simulink model "Simulink"  (R2020b)
settings: Solver=VariableStepAuto  StartTime=0.0  StopTime=11.2395  RelTol=1e-3
values from neighbouring files (symbols this model uses):
  alpha_0 = 1    [Main.m]
  b = 10    [Main.m]
  beta = 3    [Main.m]
  beta_0 = 1    [Main.m]
  c1 = rand(8,8)-0.5    [Main.m]
  c2 = rand(8,8)-0.5    [Main.m]
  c3 = rand(8,8)-0.5    [Main.m]
  c4 = rand(8,8)-0.5    [Main.m]
  delta_0 = 1    [Main.m]
  Gamma = 3    [Main.m]
  gamma = 0.1    [Main.m]
  h1_x = 5    [Main.m]
  h1_y = 5    [Main.m]
  h2_x = -5    [Main.m]
  h2_y = 5    [Main.m]
  h3_x = -5    [Main.m]
  h3_y = -5    [Main.m]
  h4_x = 5    [Main.m]
  h4_y = -5    [Main.m]
  kapa = 3    [Main.m]
  ki = diag([150,150])    [Main.m]
  kp = 20    [Main.m]
  L = full(laplacian(G))    [Main.m]
  m = 3    [Main.m]
  obs_x = 40    [Main.m]
  obs_y = 0    [Main.m]
  R = 5    [Main.m]
  r = 2    [Main.m]
  R_reg = 15    [Main.m]
  region_x = 80    [Main.m]
  region_y = 0    [Main.m]
  row_0 = 0    [Main.m]
  WL_0 = rand(number_of_neurons,1)*2    [Main.m]
  WR_0 = rand(number_of_neurons,1)*2    [Main.m]
  x1_0 = 1    [Main.m]
  x1_dot_0 = 0    [Main.m]
  x2_0 = 1    [Main.m]
  x2_dot_0 = 0    [Main.m]
  x3_0 = 1    [Main.m]
  x3_dot_0 = 0    [Main.m]
  x4_0 = 1    [Main.m]
  x4_dot_0 = 0    [Main.m]
  y1_0 = 9    [Main.m]
  y1_dot_0 = 0    [Main.m]
  y2_0 = 3    [Main.m]
  y2_dot_0 = 0    [Main.m]
  y3_0 = -3    [Main.m]
  y3_dot_0 = 0    [Main.m]
  y4_0 = -9    [Main.m]
  y4_dot_0 = 0    [Main.m]
(part 2 of 2)

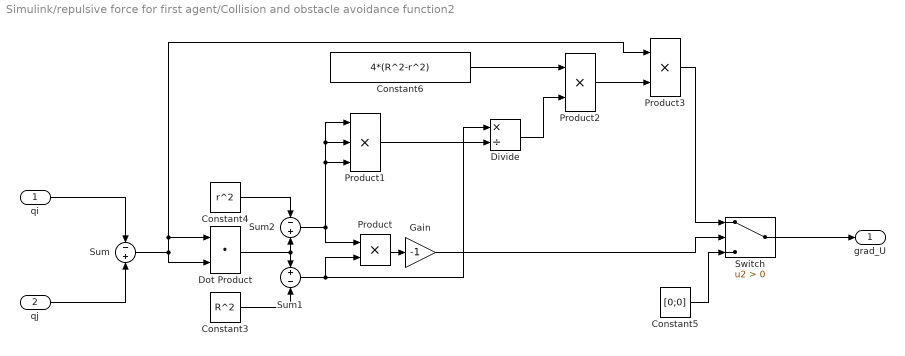
== system Simulink/repulsive force for first agent/Collision and obstacle avoidance function2 ==
  qi : Inport
  qj : Inport  Port=2
  Constant3 : Constant  Value=R^2
  Constant4 : Constant  Value=r^2
  Constant5 : Constant  Value=[0;0]
  Constant6 : Constant  Value=4*(R^2-r^2)
  Divide : Product  Inputs=*/
  Dot Product : DotProduct  InputSameDT=on  OutDataTypeStr=Inherit: Inherit via internal rule
  Gain : Gain  Gain=-1
  Product : Product
  Product1 : Product  Inputs=3
  Product2 : Product
  Product3 : Product
  Sum : Sum  Inputs=-+
  Sum1 : Sum  Inputs=+-
  Sum2 : Sum  Inputs=-+
  Switch : Switch  Criteria=u2 > Threshold
  grad_U : Outport
  wires:
  Sum1/1 -> Divide/1, Product/2
  Sum2/1 -> Product1/1, Product1/2, Product1/3, Product/1
  qi/1 -> Sum/1
  Dot Product/1 -> Sum2/2, Sum1/1
  Product1/1 -> Divide/2
  Constant5/1 -> Switch/3
  Constant4/1 -> Sum2/1
  Divide/1 -> Product2/2
  Constant3/1 -> Sum1/2
  Sum/1 -> Product3/1, Dot Product/1, Dot Product/2
  Product/1 -> Gain/1
  Gain/1 -> Switch/2
  Constant6/1 -> Product2/1
  Product3/1 -> Switch/1
  Product2/1 -> Product3/2
  Switch/1 -> grad_U/1
  qj/1 -> Sum/2

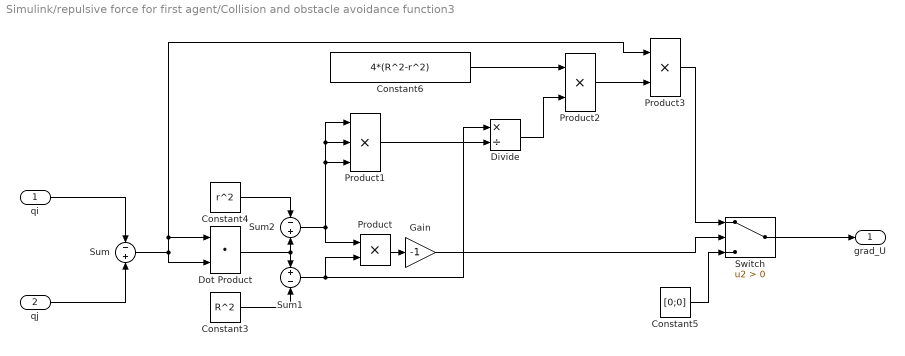
== system Simulink/repulsive force for first agent/Collision and obstacle avoidance function3 ==
  qi : Inport
  qj : Inport  Port=2
  Constant3 : Constant  Value=R^2
  Constant4 : Constant  Value=r^2
  Constant5 : Constant  Value=[0;0]
  Constant6 : Constant  Value=4*(R^2-r^2)
  Divide : Product  Inputs=*/
  Dot Product : DotProduct  InputSameDT=on  OutDataTypeStr=Inherit: Inherit via internal rule
  Gain : Gain  Gain=-1
  Product : Product
  Product1 : Product  Inputs=3
  Product2 : Product
  Product3 : Product
  Sum : Sum  Inputs=-+
  Sum1 : Sum  Inputs=+-
  Sum2 : Sum  Inputs=-+
  Switch : Switch  Criteria=u2 > Threshold
  grad_U : Outport
  wires:
  qj/1 -> Sum/2
  Switch/1 -> grad_U/1
  Product2/1 -> Product3/2
  Product3/1 -> Switch/1
  Constant6/1 -> Product2/1
  Gain/1 -> Switch/2
  Product/1 -> Gain/1
  Sum/1 -> Dot Product/2, Dot Product/1, Product3/1
  Constant3/1 -> Sum1/2
  Divide/1 -> Product2/2
  Constant4/1 -> Sum2/1
  Constant5/1 -> Switch/3
  Product1/1 -> Divide/2
  Dot Product/1 -> Sum1/1, Sum2/2
  qi/1 -> Sum/1
  Sum2/1 -> Product/1, Product1/3, Product1/2, Product1/1
  Sum1/1 -> Product/2, Divide/1

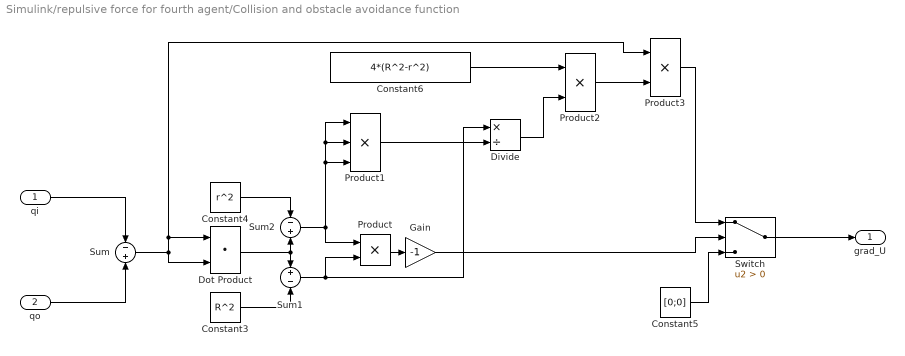
== system Simulink/repulsive force for fourth agent/Collision and obstacle avoidance function ==
  qi : Inport
  qo : Inport  Port=2
  Constant3 : Constant  Value=R^2
  Constant4 : Constant  Value=r^2
  Constant5 : Constant  Value=[0;0]
  Constant6 : Constant  Value=4*(R^2-r^2)
  Divide : Product  Inputs=*/
  Dot Product : DotProduct  InputSameDT=on  OutDataTypeStr=Inherit: Inherit via internal rule
  Gain : Gain  Gain=-1
  Product : Product
  Product1 : Product  Inputs=3
  Product2 : Product
  Product3 : Product
  Sum : Sum  Inputs=-+
  Sum1 : Sum  Inputs=+-
  Sum2 : Sum  Inputs=-+
  Switch : Switch  Criteria=u2 > Threshold
  grad_U : Outport
  wires:
  Sum1/1 -> Divide/1, Product/2
  Sum2/1 -> Product1/1, Product1/2, Product1/3, Product/1
  qi/1 -> Sum/1
  Dot Product/1 -> Sum2/2, Sum1/1
  Product1/1 -> Divide/2
  Constant5/1 -> Switch/3
  Constant4/1 -> Sum2/1
  Divide/1 -> Product2/2
  Constant3/1 -> Sum1/2
  Sum/1 -> Product3/1, Dot Product/1, Dot Product/2
  Product/1 -> Gain/1
  Gain/1 -> Switch/2
  Constant6/1 -> Product2/1
  Product3/1 -> Switch/1
  Product2/1 -> Product3/2
  Switch/1 -> grad_U/1
  qo/1 -> Sum/2

== system Simulink/repulsive force for fourth agent/Collision and obstacle avoidance function1 ==
  qi : Inport
  qj : Inport  Port=2
  Constant3 : Constant  Value=R^2
  Constant4 : Constant  Value=r^2
  Constant5 : Constant  Value=[0;0]
  Constant6 : Constant  Value=4*(R^2-r^2)
  Divide : Product  Inputs=*/
  Dot Product : DotProduct  InputSameDT=on  OutDataTypeStr=Inherit: Inherit via internal rule
  Gain : Gain  Gain=-1
  Product : Product
  Product1 : Product  Inputs=3
  Product2 : Product
  Product3 : Product
  Sum : Sum  Inputs=-+
  Sum1 : Sum  Inputs=+-
  Sum2 : Sum  Inputs=-+
  Switch : Switch  Criteria=u2 > Threshold
  grad_U : Outport
  wires:
  qj/1 -> Sum/2
  Switch/1 -> grad_U/1
  Product2/1 -> Product3/2
  Product3/1 -> Switch/1
  Constant6/1 -> Product2/1
  Gain/1 -> Switch/2
  Product/1 -> Gain/1
  Sum/1 -> Dot Product/2, Dot Product/1, Product3/1
  Constant3/1 -> Sum1/2
  Divide/1 -> Product2/2
  Constant4/1 -> Sum2/1
  Constant5/1 -> Switch/3
  Product1/1 -> Divide/2
  Dot Product/1 -> Sum1/1, Sum2/2
  qi/1 -> Sum/1
  Sum2/1 -> Product/1, Product1/3, Product1/2, Product1/1
  Sum1/1 -> Product/2, Divide/1

== system Simulink/repulsive force for fourth agent/Collision and obstacle avoidance function2 ==
  qi : Inport
  qj : Inport  Port=2
  Constant3 : Constant  Value=R^2
  Constant4 : Constant  Value=r^2
  Constant5 : Constant  Value=[0;0]
  Constant6 : Constant  Value=4*(R^2-r^2)
  Divide : Product  Inputs=*/
  Dot Product : DotProduct  InputSameDT=on  OutDataTypeStr=Inherit: Inherit via internal rule
  Gain : Gain  Gain=-1
  Product : Product
  Product1 : Product  Inputs=3
  Product2 : Product
  Product3 : Product
  Sum : Sum  Inputs=-+
  Sum1 : Sum  Inputs=+-
  Sum2 : Sum  Inputs=-+
  Switch : Switch  Criteria=u2 > Threshold
  grad_U : Outport
  wires:
  Sum1/1 -> Divide/1, Product/2
  Sum2/1 -> Product1/1, Product1/2, Product1/3, Product/1
  qi/1 -> Sum/1
  Dot Product/1 -> Sum2/2, Sum1/1
  Product1/1 -> Divide/2
  Constant5/1 -> Switch/3
  Constant4/1 -> Sum2/1
  Divide/1 -> Product2/2
  Constant3/1 -> Sum1/2
  Sum/1 -> Product3/1, Dot Product/1, Dot Product/2
  Product/1 -> Gain/1
  Gain/1 -> Switch/2
  Constant6/1 -> Product2/1
  Product3/1 -> Switch/1
  Product2/1 -> Product3/2
  Switch/1 -> grad_U/1
  qj/1 -> Sum/2

== system Simulink/repulsive force for fourth agent/Collision and obstacle avoidance function3 ==
  qi : Inport
  qj : Inport  Port=2
  Constant3 : Constant  Value=R^2
  Constant4 : Constant  Value=r^2
  Constant5 : Constant  Value=[0;0]
  Constant6 : Constant  Value=4*(R^2-r^2)
  Divide : Product  Inputs=*/
  Dot Product : DotProduct  InputSameDT=on  OutDataTypeStr=Inherit: Inherit via internal rule
  Gain : Gain  Gain=-1
  Product : Product
  Product1 : Product  Inputs=3
  Product2 : Product
  Product3 : Product
  Sum : Sum  Inputs=-+
  Sum1 : Sum  Inputs=+-
  Sum2 : Sum  Inputs=-+
  Switch : Switch  Criteria=u2 > Threshold
  grad_U : Outport
  wires:
  qj/1 -> Sum/2
  Switch/1 -> grad_U/1
  Product2/1 -> Product3/2
  Product3/1 -> Switch/1
  Constant6/1 -> Product2/1
  Gain/1 -> Switch/2
  Product/1 -> Gain/1
  Sum/1 -> Dot Product/2, Dot Product/1, Product3/1
  Constant3/1 -> Sum1/2
  Divide/1 -> Product2/2
  Constant4/1 -> Sum2/1
  Constant5/1 -> Switch/3
  Product1/1 -> Divide/2
  Dot Product/1 -> Sum1/1, Sum2/2
  qi/1 -> Sum/1
  Sum2/1 -> Product/1, Product1/3, Product1/2, Product1/1
  Sum1/1 -> Product/2, Divide/1

== system Simulink/repulsive force for second agent/Collision and obstacle avoidance function ==
  qi : Inport
  qo : Inport  Port=2
  Constant3 : Constant  Value=R^2
  Constant4 : Constant  Value=r^2
  Constant5 : Constant  Value=[0;0]
  Constant6 : Constant  Value=4*(R^2-r^2)
  Divide : Product  Inputs=*/
  Dot Product : DotProduct  InputSameDT=on  OutDataTypeStr=Inherit: Inherit via internal rule
  Gain : Gain  Gain=-1
  Product : Product
  Product1 : Product  Inputs=3
  Product2 : Product
  Product3 : Product
  Sum : Sum  Inputs=-+
  Sum1 : Sum  Inputs=+-
  Sum2 : Sum  Inputs=-+
  Switch : Switch  Criteria=u2 > Threshold
  grad_U : Outport
  wires:
  qo/1 -> Sum/2
  Switch/1 -> grad_U/1
  Product2/1 -> Product3/2
  Product3/1 -> Switch/1
  Constant6/1 -> Product2/1
  Gain/1 -> Switch/2
  Product/1 -> Gain/1
  Sum/1 -> Dot Product/2, Dot Product/1, Product3/1
  Constant3/1 -> Sum1/2
  Divide/1 -> Product2/2
  Constant4/1 -> Sum2/1
  Constant5/1 -> Switch/3
  Product1/1 -> Divide/2
  Dot Product/1 -> Sum1/1, Sum2/2
  qi/1 -> Sum/1
  Sum2/1 -> Product/1, Product1/3, Product1/2, Product1/1
  Sum1/1 -> Product/2, Divide/1

== system Simulink/repulsive force for second agent/Collision and obstacle avoidance function1 ==
  qi : Inport
  qj : Inport  Port=2
  Constant3 : Constant  Value=R^2
  Constant4 : Constant  Value=r^2
  Constant5 : Constant  Value=[0;0]
  Constant6 : Constant  Value=4*(R^2-r^2)
  Divide : Product  Inputs=*/
  Dot Product : DotProduct  InputSameDT=on  OutDataTypeStr=Inherit: Inherit via internal rule
  Gain : Gain  Gain=-1
  Product : Product
  Product1 : Product  Inputs=3
  Product2 : Product
  Product3 : Product
  Sum : Sum  Inputs=-+
  Sum1 : Sum  Inputs=+-
  Sum2 : Sum  Inputs=-+
  Switch : Switch  Criteria=u2 > Threshold
  grad_U : Outport
  wires:
  Sum1/1 -> Divide/1, Product/2
  Sum2/1 -> Product1/1, Product1/2, Product1/3, Product/1
  qi/1 -> Sum/1
  Dot Product/1 -> Sum2/2, Sum1/1
  Product1/1 -> Divide/2
  Constant5/1 -> Switch/3
  Constant4/1 -> Sum2/1
  Divide/1 -> Product2/2
  Constant3/1 -> Sum1/2
  Sum/1 -> Product3/1, Dot Product/1, Dot Product/2
  Product/1 -> Gain/1
  Gain/1 -> Switch/2
  Constant6/1 -> Product2/1
  Product3/1 -> Switch/1
  Product2/1 -> Product3/2
  Switch/1 -> grad_U/1
  qj/1 -> Sum/2

== system Simulink/repulsive force for second agent/Collision and obstacle avoidance function2 ==
  qi : Inport
  qj : Inport  Port=2
  Constant3 : Constant  Value=R^2
  Constant4 : Constant  Value=r^2
  Constant5 : Constant  Value=[0;0]
  Constant6 : Constant  Value=4*(R^2-r^2)
  Divide : Product  Inputs=*/
  Dot Product : DotProduct  InputSameDT=on  OutDataTypeStr=Inherit: Inherit via internal rule
  Gain : Gain  Gain=-1
  Product : Product
  Product1 : Product  Inputs=3
  Product2 : Product
  Product3 : Product
  Sum : Sum  Inputs=-+
  Sum1 : Sum  Inputs=+-
  Sum2 : Sum  Inputs=-+
  Switch : Switch  Criteria=u2 > Threshold
  grad_U : Outport
  wires:
  qj/1 -> Sum/2
  Switch/1 -> grad_U/1
  Product2/1 -> Product3/2
  Product3/1 -> Switch/1
  Constant6/1 -> Product2/1
  Gain/1 -> Switch/2
  Product/1 -> Gain/1
  Sum/1 -> Dot Product/2, Dot Product/1, Product3/1
  Constant3/1 -> Sum1/2
  Divide/1 -> Product2/2
  Constant4/1 -> Sum2/1
  Constant5/1 -> Switch/3
  Product1/1 -> Divide/2
  Dot Product/1 -> Sum1/1, Sum2/2
  qi/1 -> Sum/1
  Sum2/1 -> Product/1, Product1/3, Product1/2, Product1/1
  Sum1/1 -> Product/2, Divide/1

== system Simulink/repulsive force for second agent/Collision and obstacle avoidance function3 ==
  qi : Inport
  qj : Inport  Port=2
  Constant3 : Constant  Value=R^2
  Constant4 : Constant  Value=r^2
  Constant5 : Constant  Value=[0;0]
  Constant6 : Constant  Value=4*(R^2-r^2)
  Divide : Product  Inputs=*/
  Dot Product : DotProduct  InputSameDT=on  OutDataTypeStr=Inherit: Inherit via internal rule
  Gain : Gain  Gain=-1
  Product : Product
  Product1 : Product  Inputs=3
  Product2 : Product
  Product3 : Product
  Sum : Sum  Inputs=-+
  Sum1 : Sum  Inputs=+-
  Sum2 : Sum  Inputs=-+
  Switch : Switch  Criteria=u2 > Threshold
  grad_U : Outport
  wires:
  Sum1/1 -> Divide/1, Product/2
  Sum2/1 -> Product1/1, Product1/2, Product1/3, Product/1
  qi/1 -> Sum/1
  Dot Product/1 -> Sum2/2, Sum1/1
  Product1/1 -> Divide/2
  Constant5/1 -> Switch/3
  Constant4/1 -> Sum2/1
  Divide/1 -> Product2/2
  Constant3/1 -> Sum1/2
  Sum/1 -> Product3/1, Dot Product/1, Dot Product/2
  Product/1 -> Gain/1
  Gain/1 -> Switch/2
  Constant6/1 -> Product2/1
  Product3/1 -> Switch/1
  Product2/1 -> Product3/2
  Switch/1 -> grad_U/1
  qj/1 -> Sum/2

== system Simulink/repulsive force for third agent/Collision and obstacle avoidance function ==
  qi : Inport
  qo : Inport  Port=2
  Constant3 : Constant  Value=R^2
  Constant4 : Constant  Value=r^2
  Constant5 : Constant  Value=[0;0]
  Constant6 : Constant  Value=4*(R^2-r^2)
  Divide : Product  Inputs=*/
  Dot Product : DotProduct  InputSameDT=on  OutDataTypeStr=Inherit: Inherit via internal rule
  Gain : Gain  Gain=-1
  Product : Product
  Product1 : Product  Inputs=3
  Product2 : Product
  Product3 : Product
  Sum : Sum  Inputs=-+
  Sum1 : Sum  Inputs=+-
  Sum2 : Sum  Inputs=-+
  Switch : Switch  Criteria=u2 > Threshold
  grad_U : Outport
  wires:
  qo/1 -> Sum/2
  Switch/1 -> grad_U/1
  Product2/1 -> Product3/2
  Product3/1 -> Switch/1
  Constant6/1 -> Product2/1
  Gain/1 -> Switch/2
  Product/1 -> Gain/1
  Sum/1 -> Dot Product/2, Dot Product/1, Product3/1
  Constant3/1 -> Sum1/2
  Divide/1 -> Product2/2
  Constant4/1 -> Sum2/1
  Constant5/1 -> Switch/3
  Product1/1 -> Divide/2
  Dot Product/1 -> Sum1/1, Sum2/2
  qi/1 -> Sum/1
  Sum2/1 -> Product/1, Product1/3, Product1/2, Product1/1
  Sum1/1 -> Product/2, Divide/1

== system Simulink/repulsive force for third agent/Collision and obstacle avoidance function1 ==
  qi : Inport
  qj : Inport  Port=2
  Constant3 : Constant  Value=R^2
  Constant4 : Constant  Value=r^2
  Constant5 : Constant  Value=[0;0]
  Constant6 : Constant  Value=4*(R^2-r^2)
  Divide : Product  Inputs=*/
  Dot Product : DotProduct  InputSameDT=on  OutDataTypeStr=Inherit: Inherit via internal rule
  Gain : Gain  Gain=-1
  Product : Product
  Product1 : Product  Inputs=3
  Product2 : Product
  Product3 : Product
  Sum : Sum  Inputs=-+
  Sum1 : Sum  Inputs=+-
  Sum2 : Sum  Inputs=-+
  Switch : Switch  Criteria=u2 > Threshold
  grad_U : Outport
  wires:
  Sum1/1 -> Divide/1, Product/2
  Sum2/1 -> Product1/1, Product1/2, Product1/3, Product/1
  qi/1 -> Sum/1
  Dot Product/1 -> Sum2/2, Sum1/1
  Product1/1 -> Divide/2
  Constant5/1 -> Switch/3
  Constant4/1 -> Sum2/1
  Divide/1 -> Product2/2
  Constant3/1 -> Sum1/2
  Sum/1 -> Product3/1, Dot Product/1, Dot Product/2
  Product/1 -> Gain/1
  Gain/1 -> Switch/2
  Constant6/1 -> Product2/1
  Product3/1 -> Switch/1
  Product2/1 -> Product3/2
  Switch/1 -> grad_U/1
  qj/1 -> Sum/2

== system Simulink/repulsive force for third agent/Collision and obstacle avoidance function2 ==
  qi : Inport
  qj : Inport  Port=2
  Constant3 : Constant  Value=R^2
  Constant4 : Constant  Value=r^2
  Constant5 : Constant  Value=[0;0]
  Constant6 : Constant  Value=4*(R^2-r^2)
  Divide : Product  Inputs=*/
  Dot Product : DotProduct  InputSameDT=on  OutDataTypeStr=Inherit: Inherit via internal rule
  Gain : Gain  Gain=-1
  Product : Product
  Product1 : Product  Inputs=3
  Product2 : Product
  Product3 : Product
  Sum : Sum  Inputs=-+
  Sum1 : Sum  Inputs=+-
  Sum2 : Sum  Inputs=-+
  Switch : Switch  Criteria=u2 > Threshold
  grad_U : Outport
  wires:
  qj/1 -> Sum/2
  Switch/1 -> grad_U/1
  Product2/1 -> Product3/2
  Product3/1 -> Switch/1
  Constant6/1 -> Product2/1
  Gain/1 -> Switch/2
  Product/1 -> Gain/1
  Sum/1 -> Dot Product/2, Dot Product/1, Product3/1
  Constant3/1 -> Sum1/2
  Divide/1 -> Product2/2
  Constant4/1 -> Sum2/1
  Constant5/1 -> Switch/3
  Product1/1 -> Divide/2
  Dot Product/1 -> Sum1/1, Sum2/2
  qi/1 -> Sum/1
  Sum2/1 -> Product/1, Product1/3, Product1/2, Product1/1
  Sum1/1 -> Product/2, Divide/1

== system Simulink/repulsive force for third agent/Collision and obstacle avoidance function3 ==
  qi : Inport
  qj : Inport  Port=2
  Constant3 : Constant  Value=R^2
  Constant4 : Constant  Value=r^2
  Constant5 : Constant  Value=[0;0]
  Constant6 : Constant  Value=4*(R^2-r^2)
  Divide : Product  Inputs=*/
  Dot Product : DotProduct  InputSameDT=on  OutDataTypeStr=Inherit: Inherit via internal rule
  Gain : Gain  Gain=-1
  Product : Product
  Product1 : Product  Inputs=3
  Product2 : Product
  Product3 : Product
  Sum : Sum  Inputs=-+
  Sum1 : Sum  Inputs=+-
  Sum2 : Sum  Inputs=-+
  Switch : Switch  Criteria=u2 > Threshold
  grad_U : Outport
  wires:
  Sum1/1 -> Divide/1, Product/2
  Sum2/1 -> Product1/1, Product1/2, Product1/3, Product/1
  qi/1 -> Sum/1
  Dot Product/1 -> Sum2/2, Sum1/1
  Product1/1 -> Divide/2
  Constant5/1 -> Switch/3
  Constant4/1 -> Sum2/1
  Divide/1 -> Product2/2
  Constant3/1 -> Sum1/2
  Sum/1 -> Product3/1, Dot Product/1, Dot Product/2
  Product/1 -> Gain/1
  Gain/1 -> Switch/2
  Constant6/1 -> Product2/1
  Product3/1 -> Switch/1
  Product2/1 -> Product3/2
  Switch/1 -> grad_U/1
  qj/1 -> Sum/2

== system Simulink/s and x signals for first agent/qri_dot ==
  e : Inport
  alpha : Inport  Port=2
  beta : Inport  Port=3
  neg_deta_xi : Inport  Port=4
  Product : Product
  Product1 : Product
  Sum : Sum  Inputs=-+
  qri_dot : Outport
  wires:
  e/1 -> Product/1
  neg_deta_xi/1 -> Product1/2
  Product/1 -> Sum/1
  Sum/1 -> qri_dot/1
  alpha/1 -> Product/2
  Product1/1 -> Sum/2
  beta/1 -> Product1/1

== system Simulink/s and x signals for first agent/qri_dot_dot ==
  e : Inport
  alpha : Inport  Port=2
  beta : Inport  Port=3
  neg_deta_xi : Inport  Port=4
  e_dot : Inport  Port=5
  alpha_dot : Inport  Port=6
  beta_dot : Inport  Port=7
  neg_deta_xi_dot : Inport  Port=8
  Product{,1..3} (4 alike) : Product
  Sum : Sum  Inputs=--++
  qri_dot_dot : Outport
  wires:
  Sum/1 -> qri_dot_dot/1
  e/1 -> Product/1
  alpha_dot/1 -> Product/2
  alpha/1 -> Product1/1
  e_dot/1 -> Product1/2
  beta/1 -> Product2/1
  neg_deta_xi_dot/1 -> Product2/2
  neg_deta_xi/1 -> Product3/1
  beta_dot/1 -> Product3/2
  Product/1 -> Sum/1
  Product3/1 -> Sum/4
  Product1/1 -> Sum/2
  Product2/1 -> Sum/3

== system Simulink/s and x signals for fourth agent/qri_dot ==
  e : Inport
  alpha : Inport  Port=2
  beta : Inport  Port=3
  neg_deta_xi : Inport  Port=4
  Product : Product
  Product1 : Product
  Sum : Sum  Inputs=-+
  qri_dot : Outport
  wires:
  beta/1 -> Product1/1
  Product1/1 -> Sum/2
  alpha/1 -> Product/2
  Sum/1 -> qri_dot/1
  Product/1 -> Sum/1
  neg_deta_xi/1 -> Product1/2
  e/1 -> Product/1

== system Simulink/s and x signals for fourth agent/qri_dot_dot ==
  e : Inport
  alpha : Inport  Port=2
  beta : Inport  Port=3
  neg_deta_xi : Inport  Port=4
  e_dot : Inport  Port=5
  alpha_dot : Inport  Port=6
  beta_dot : Inport  Port=7
  neg_deta_xi_dot : Inport  Port=8
  Product{,1..3} (4 alike) : Product
  Sum : Sum  Inputs=--++
  qri_dot_dot : Outport
  wires:
  Product2/1 -> Sum/3
  Product1/1 -> Sum/2
  Product3/1 -> Sum/4
  Product/1 -> Sum/1
  beta_dot/1 -> Product3/2
  neg_deta_xi/1 -> Product3/1
  neg_deta_xi_dot/1 -> Product2/2
  beta/1 -> Product2/1
  e_dot/1 -> Product1/2
  alpha/1 -> Product1/1
  alpha_dot/1 -> Product/2
  e/1 -> Product/1
  Sum/1 -> qri_dot_dot/1

== system Simulink/s and x signals for second agent/qri_dot ==
  e : Inport
  alpha : Inport  Port=2
  beta : Inport  Port=3
  neg_deta_xi : Inport  Port=4
  Product : Product
  Product1 : Product
  Sum : Sum  Inputs=-+
  qri_dot : Outport
  wires:
  beta/1 -> Product1/1
  Product1/1 -> Sum/2
  alpha/1 -> Product/2
  Sum/1 -> qri_dot/1
  Product/1 -> Sum/1
  neg_deta_xi/1 -> Product1/2
  e/1 -> Product/1

== system Simulink/s and x signals for second agent/qri_dot_dot ==
  e : Inport
  alpha : Inport  Port=2
  beta : Inport  Port=3
  neg_deta_xi : Inport  Port=4
  e_dot : Inport  Port=5
  alpha_dot : Inport  Port=6
  beta_dot : Inport  Port=7
  neg_deta_xi_dot : Inport  Port=8
  Product{,1..3} (4 alike) : Product
  Sum : Sum  Inputs=--++
  qri_dot_dot : Outport
  wires:
  Product2/1 -> Sum/3
  Product1/1 -> Sum/2
  Product3/1 -> Sum/4
  Product/1 -> Sum/1
  beta_dot/1 -> Product3/2
  neg_deta_xi/1 -> Product3/1
  neg_deta_xi_dot/1 -> Product2/2
  beta/1 -> Product2/1
  e_dot/1 -> Product1/2
  alpha/1 -> Product1/1
  alpha_dot/1 -> Product/2
  e/1 -> Product/1
  Sum/1 -> qri_dot_dot/1

== system Simulink/s and x signals for third agent/qri_dot ==
  e : Inport
  alpha : Inport  Port=2
  beta : Inport  Port=3
  neg_deta_xi : Inport  Port=4
  Product : Product
  Product1 : Product
  Sum : Sum  Inputs=-+
  qri_dot : Outport
  wires:
  e/1 -> Product/1
  neg_deta_xi/1 -> Product1/2
  Product/1 -> Sum/1
  Sum/1 -> qri_dot/1
  alpha/1 -> Product/2
  Product1/1 -> Sum/2
  beta/1 -> Product1/1

== system Simulink/s and x signals for third agent/qri_dot_dot ==
  e : Inport
  alpha : Inport  Port=2
  beta : Inport  Port=3
  neg_deta_xi : Inport  Port=4
  e_dot : Inport  Port=5
  alpha_dot : Inport  Port=6
  beta_dot : Inport  Port=7
  neg_deta_xi_dot : Inport  Port=8
  Product{,1..3} (4 alike) : Product
  Sum : Sum  Inputs=--++
  qri_dot_dot : Outport
  wires:
  Sum/1 -> qri_dot_dot/1
  e/1 -> Product/1
  alpha_dot/1 -> Product/2
  alpha/1 -> Product1/1
  e_dot/1 -> Product1/2
  beta/1 -> Product2/1
  neg_deta_xi_dot/1 -> Product2/2
  neg_deta_xi/1 -> Product3/1
  beta_dot/1 -> Product3/2
  Product/1 -> Sum/1
  Product3/1 -> Sum/4
  Product1/1 -> Sum/2
  Product2/1 -> Sum/3
